simulink model "counter"  (R2020a)
settings: Solver=VariableStepAuto  StartTime=0.0  StopTime=10.0  RelTol=1e-3
settings Model: Creator=Admin  LastModifiedBy=Admin

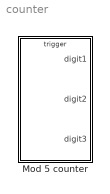
== system counter ==
  Mod 5 counter : Stateflow chart  TreatAsAtomicUnit=on

== stateflow chart counter/Mod 5 counter ==
  settings: executeAtInitialization=1
  state Digit_one [parallel]
    settings: executionOrder=1
    state state_zero
      entry: digit1=0;
    state state_one
      entry: digit1=1;
    state state_two
      entry: digit1=2;
    state state_four
      entry: digit1=4;
    state state_three
      entry: digit1=3;
    (default) -> Digit_one.state_zero
    Digit_one.state_zero -> Digit_one.state_one : event1
    Digit_one.state_one -> Digit_one.state_two : event1
    Digit_one.state_four -> Digit_one.state_zero : event1/{event2}
    Digit_one.state_two -> Digit_one.state_three : event1
    Digit_one.state_three -> Digit_one.state_four : event1
  state Digit_two [parallel]
    settings: executionOrder=2
    state state_zero
      entry: digit2=0;
    state state_one
      entry: digit2=1;
    state state_two
      entry: digit2=2;
    state state_four
      entry: digit2=4;
    state state_three
      entry: digit2=3;
    (default) -> Digit_two.state_zero
    Digit_two.state_zero -> Digit_two.state_one : event2
    Digit_two.state_one -> Digit_two.state_two : event2
    Digit_two.state_four -> Digit_two.state_zero : event2/{event3}
    Digit_two.state_two -> Digit_two.state_three : event2
    Digit_two.state_three -> Digit_two.state_four : event2
  state Digit_three [parallel]
    settings: executionOrder=3
    state state_zero
      entry: digit3=0;
    state state_one
      entry: digit3=1;
    state state_two
      entry: digit3=2;
    state state_four
      entry: digit3=4;
    state state_three
      entry: digit3=3;
    (default) -> Digit_three.state_zero
    Digit_three.state_zero -> Digit_three.state_one : event3
    Digit_three.state_one -> Digit_three.state_two : event3
    Digit_three.state_four -> Digit_three.state_zero : event3
    Digit_three.state_two -> Digit_three.state_three : event3
    Digit_three.state_three -> Digit_three.state_four : event3
  data: digit1 output; digit2 output; digit3 output
  events: event2 local FUNCTION_CALL_EVENT; event3 local FUNCTION_CALL_EVENT; event1 input RISING_EDGE_EVENT
